simulink model "FABRIK_Simulation"  (R2019a)
settings: Solver=FixedStepAuto  StartTime=0.0  StopTime=1  FixedStep=0.01  RelTol=1e-3
settings Model: Creator=Admin  LastModifiedBy=Admin

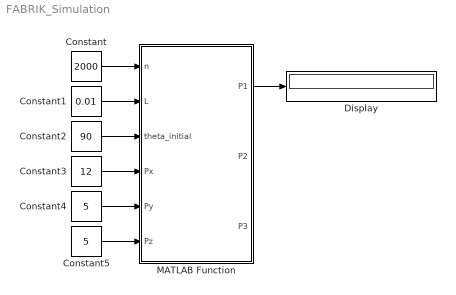
== system FABRIK_Simulation ==
  Constant : Constant  Value=2000
  Constant1 : Constant  Value=0.01
  Constant2 : Constant  Value=90
  Constant3 : Constant  Value=12
  Constant4 : Constant  Value=5
  Constant5 : Constant  Value=5
  Display : Display
  MATLAB Function : MATLAB Function  TreatAsAtomicUnit=on
  wires:
  Constant/1 -> MATLAB Function/1(n)
  Constant1/1 -> MATLAB Function/2(L)
  Constant2/1 -> MATLAB Function/3(theta_initial)
  MATLAB Function/1(P1) -> Display/1
  Constant3/1 -> MATLAB Function/4(Px)
  Constant4/1 -> MATLAB Function/5(Py)
  Constant5/1 -> MATLAB Function/6(Pz)

== matlab function FABRIK_Simulation/MATLAB Function ==
  data: n input; P1 output; L input; theta_initial input; Px input; P2 output; P3 output; Py input; Pz input
function [P1,P2,P3]= fcn(n,L,theta_initial,Px,Py,Pz)
    theta = zeros(n,1);
    t = [Px Py Pz];
    theta(1,1) = theta_initial;
    P = Tao_Robot_n_diem(n,L,theta);
    P = FABRIK(L,n,P,t);
    P1 = 0;
    P2 = 0;
    P3 = 0;
end
